simulink model "Problem9"  (R2020a)
settings: Solver=VariableStepAuto  StartTime=0.0  StopTime=20.0  RelTol=1e-3
libraries: simulink_extras x2
settings Model: Creator=HP  LastModifiedBy=HP

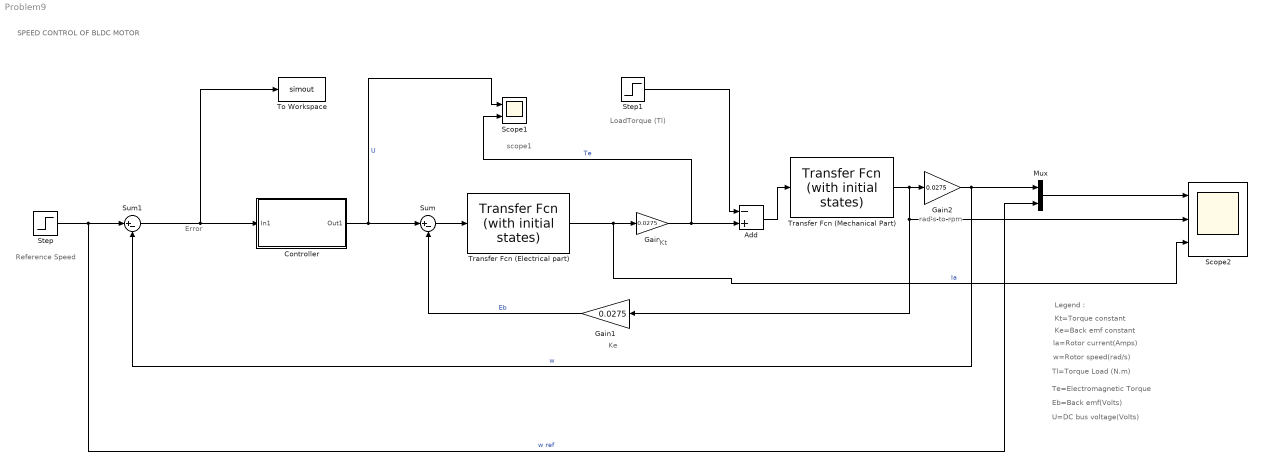
== system Problem9 ==
  note: SPEED CONTROL OF BLDC MOTOR
  note: rad's to rpm
  note: Ke
  note: Kt
  note: LoadTorque
      |      (Tl)
  note: scope1
  note: Error
  note: Reference Speed
  note: Legend :
  note: la=Rotor current(Amps)
  note: Ke=Back emf constant
  note: Te=Electromagnetic Torque
  note: w=Rotor speed(rad/s)
  note: Eb=Back emf(Volts)
  note: Kt=Torque constant
  note: Tl=Torque Load (N.m)
  note: U=DC bus voltage(Volts)
  Add : Sum  Inputs=-+
  Controller : Subsystem
  Gain : Gain  Gain=0.0275
  Gain1 : Gain  Gain=0.0275
  Gain2 : Gain  Gain=0.0275
  Mux : Mux  Inputs=2
  Scope1 : Scope  NumInputPorts=2
  Scope2 : Scope  NumInputPorts=3
  Step : Step  After=1500  SampleTime=0
  Step1 : Step  Time=0.1  After=10  SampleTime=0
  Sum : Sum  Inputs=|+-
  Sum1 : Sum  Inputs=|+-
  To Workspace : ToWorkspace  VariableName=simout  SaveFormat=Timeseries  SampleTime=-1
  Transfer Fcn (Electrical part) : simulink_extras/Additional Linear/Transfer Fcn (with initial states)  N=[1]  D="[0.0001  0.014]"  X0=.5
  Transfer Fcn (Mechanical Part) : simulink_extras/Additional Linear/Transfer Fcn (with initial states)  N=[1]  D="[0.0002  0.004586]"  X0=.5
  wires:
  Gain1/1 -> Sum/2  "Eb"
  Controller/1(Out1) -> Scope1/1, Sum/1  "U"
  Sum1/1 -> To Workspace/1, Controller/1(In1)
  Sum/1 -> Transfer Fcn (Electrical part)/1
  Transfer Fcn (Electrical part)/1 -> Gain/1, Scope2/3  "Ia"
  Gain/1 -> Scope1/2, Add/2  "Te"
  Add/1 -> Transfer Fcn (Mechanical Part)/1
  Step1/1 -> Add/1
  Transfer Fcn (Mechanical Part)/1 -> Gain1/1, Scope2/2, Gain2/1
  Step/1 -> Mux/2, Sum1/1  "w ref"
  Mux/1 -> Scope2/1
  Gain2/1 -> Sum1/2, Mux/1  "w"

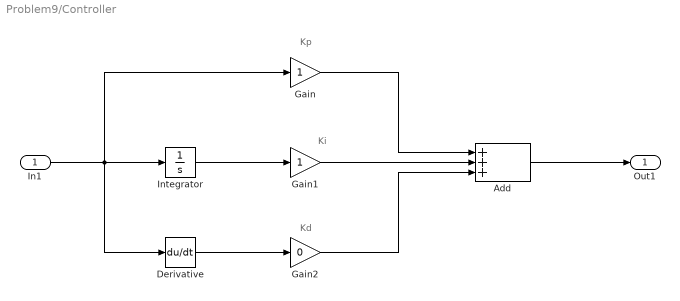
== system Problem9/Controller ==
  note: Kd
  note: Ki
  note: Kp
  In1 : Inport
  Add : Sum  Inputs=+++
  Derivative : Derivative
  Gain : Gain
  Gain1 : Gain
  Gain2 : Gain  Gain=0
  Integrator : Integrator
  Out1 : Outport
  wires:
  Add/1 -> Out1/1
  In1/1 -> Gain/1, Derivative/1, Integrator/1
  Integrator/1 -> Gain1/1
  Gain1/1 -> Add/2
  Gain2/1 -> Add/3
  Gain/1 -> Add/1
  Derivative/1 -> Gain2/1
